simulink model "AM"  (R2019b)
settings: Solver=VariableStepAuto  StartTime=0.0  StopTime=10.0  RelTol=1e-3
libraries: commanapbnd3 x2, eeGeneralControl x2
settings Model: Creator=Win 10  LastModifiedBy=thuma

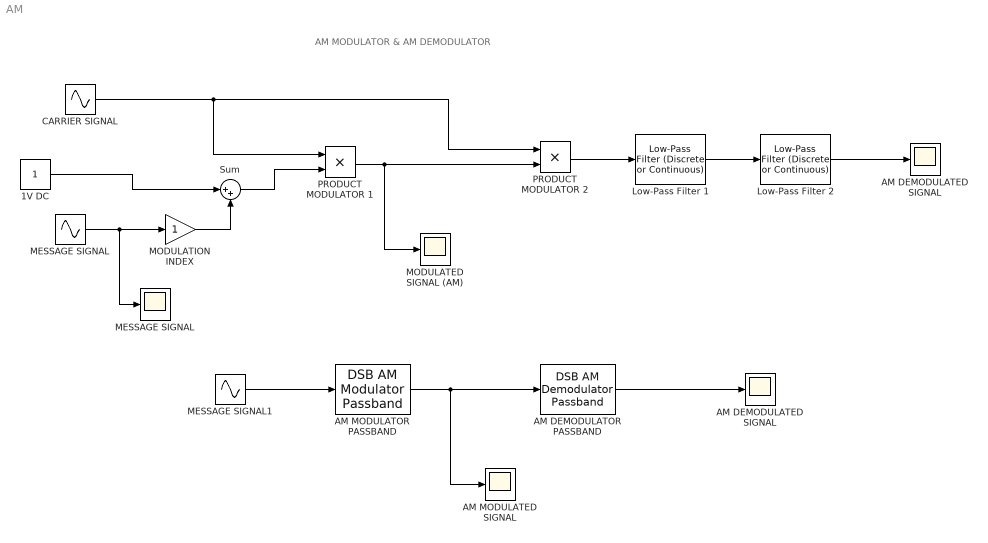
== system AM ==
  note: AM MODULATOR & AM DEMODULATOR
  " AM DEMODULATOR PASSBAND" : commanapbnd3/DSB AM Demodulator Passband  Fc=20  Ph=0  method=Butterworth  n=8  cf=18  Rp=0.1  Rs=50  Offset=0
      settings: SourceProductName=Communications Toolbox  SourceProductBaseCode=CM
  " AM DEMODULATED SIGNAL " : Scope
  " AM MODULATED SIGNAL " : Scope
  " AM MODULATOR PASSBAND " : commanapbnd3/DSB AM Modulator Passband  Fc=20  Ph=0  Offset=0
      settings: SourceProductName=Communications Toolbox  SourceProductBaseCode=CM
  " Low-Pass Filter 1" : eeGeneralControl/Low-Pass Filter (Discrete or Continuous)  K=2  T=1  B=10  A=-10  Ts=0
      settings: SourceProductName=Simscape Electrical
  " Low-Pass Filter 2" : eeGeneralControl/Low-Pass Filter (Discrete or Continuous)  K=10  T=1  B=50  A=-50  Ts=0
      settings: SourceProductName=Simscape Electrical
  1V DC : Constant
  AM DEMODULATED SIGNAL : Scope
  CARRIER SIGNAL : Sin  Frequency=2*pi*5  SampleTime=0.001
  MESSAGE SIGNAL : Sin  Frequency=2*pi*1  SampleTime=0.001
  MESSAGE SIGNAL1 : Sin  Frequency=2*pi*1  SampleTime=0.001
  MESSAGE SIGNAL : Scope
  MODULATED SIGNAL (AM) : Scope
  "MODULATION INDEX " : Gain
  PRODUCT MODULATOR 1 : Product
  PRODUCT MODULATOR 2 : Product
  Sum : Sum  Inputs=|++
  wires:
  1V DC/1 -> Sum/1
  MESSAGE SIGNAL/1 -> MESSAGE SIGNAL/1, "MODULATION INDEX "/1
  "MODULATION INDEX "/1 -> Sum/2
  PRODUCT MODULATOR 1/1 -> MODULATED SIGNAL (AM)/1, PRODUCT MODULATOR 2/2
  PRODUCT MODULATOR 2/1 -> " Low-Pass Filter 1"/1
  " AM DEMODULATOR PASSBAND"/1 -> " AM DEMODULATED SIGNAL "/1
  " AM MODULATOR PASSBAND "/1 -> " AM MODULATED SIGNAL "/1, " AM DEMODULATOR PASSBAND"/1
  MESSAGE SIGNAL1/1 -> " AM MODULATOR PASSBAND "/1
  " Low-Pass Filter 2"/1 -> AM DEMODULATED SIGNAL/1
  " Low-Pass Filter 1"/1 -> " Low-Pass Filter 2"/1
  CARRIER SIGNAL/1 -> PRODUCT MODULATOR 2/1, PRODUCT MODULATOR 1/1
  Sum/1 -> PRODUCT MODULATOR 1/2
